simulink model "M10B39_es_V1"  (R2024b)
settings: Solver=ode23tb  StartTime=0.0  StopTime=20  FixedStep=0.001  RelTol=1e-3  EnableMultiTasking=on
InitFcn:
  | initAll;
values from neighbouring files (symbols this model uses):
  acom = 100    [initAll_V1.m]    (also in initAll_V2.m; initAll_V3.m; parameterinit.mat)
  AVm0 = [4.26082678503 4.656135219]    [parameterinit.mat]
  bcom = 50    [initAll_V1.m]    (also in initAll_V2.m; initAll_V3.m; parameterinit.mat)
  commun = 0*commun    [initAll_V1.m]    (also in initAll_V2.m; initAll_V3.m; parameterinit.mat = [0  0  0; 0  0  0; 0  0  0; 0  0  0])
  DataDelay = 0.0*DataDelay    [initAll_V1.m]    (also in initAll_V2.m; initAll_V3.m; parameterinit.mat = [0  0  0; 0  0  0; 0  0  0; 0  0  0])
  ESinit =     [parameterinit.mat]
  fB = 50    [initAll.m]    (also in initAll_V1.m; initAll_V2.m; initAll_V3.m; parameterinit.mat)
  Geninit = Generator_init(opdata,SynMach_in_gidx)    [initAll.m]    (also in initAll_V1.m; initAll_V2.m; initAll_V3.m = Generator_init(opdata_all,SynMach_in_gidx1); parameterinit.mat = )
  lam = 100    [initAll_V1.m]    (also in initAll_V2.m; initAll_V3.m; parameterinit.mat)
  SgridB = 100    [initAll.m]    (also in initAll_V1.m; initAll_V2.m; initAll_V3.m; parameterinit.mat)
  wB = 2*pi*fB    (= 314.159265359)    [initAll.m]    (also in initAll_V1.m; initAll_V2.m; initAll_V3.m; parameterinit.mat)
  Windinit =     [parameterinit.mat]
  YY_load = [3.65450097002 -2.05705688056 0 0 0 0 0 0 0 0 0 0 ... (1521 elements, 39x39)]    [parameterinit.mat]    (also in powerflowcaculate.m = full(YY))
undefined symbols (not defined in the file or in its folder): c1, c2, c3, c4, c5, c6, cp_nom, lambda_nom, P_wind_base, Pelec_base, Pnom
libraries: spsBistableLib x12, simulink_extras x4, slpidlib x1, simulink x1
(part 1 of 7)
settings Model: Creator=m  LastModifiedBy=86182
settings SolverCC: AlgebraicLoopSolver=TrustRegion
settings DataIOCC: SignalLoggingSaveFormat=ModelDataLogs  DSMLogging=off  ReturnWorkspaceOutputs=off  SignalLoggingName=logout
settings OptimizationCC: ExpressionDepthLimit=2147483647  LifeSpan=inf
settings DebuggingCC: SaveWithParameterizedLinksMsg=none  UnderspecifiedInitializationDetection=Classic  MergeDetectMultiDrivingBlocksExec=none  SignalResolutionControl=TryResolveAllWithWarning  MultiTaskDSMMsg=warning  MultiTaskCondExecSysMsg=none  FcnCallInpInsideContextMsg=warning  UnconnectedInputMsg=warning  UnconnectedOutputMsg=warning  UnconnectedLineMsg=warning  StateNameClashWarn=warning  SFUnexpectedBacktrackingDiag=warning  SFNoUnconditionalDefaultTransitionDiag=warning  SFExecutionAtInitializationDiag=none  ArithmeticOperatorsInVariantConditions=warning
settings HardwareCC: ProdBitPerPointer=32  ProdBitPerSizeT=32  ProdBitPerPtrDiffT=32  ProdLargestAtomicFloat=None  ProdIntDivRoundTo=Undefined  ProdEndianess=Unspecified  ProdWordSize=32  ProdHWDeviceType=32-bit Generic  TargetUnknown=on
settings ModelReferenceCC: EnableRefExpFcnMdlSchedulingChecks=on  PropagateSignalLabelsOutOfModel=off
settings SFSimCC: SimUseLocalCustomCode=off  CustomCodeUndefinedFunction=UseInterfaceOnly
settings RTWCC: RTWUseLocalCustomCode=off  GPUComputeCapability=3.5  DLArmComputeVersion=19.05
settings CodeAppCC: StateflowObjectComments=on
settings GRTTargetCC: TargetLangStandard=C89/C90 (ANSI)  CombineOutputUpdateFcns=off  GRTInterface=on
settings ConfigComp: CovMetricSettings=dw  CovSaveCumulativeToWorkspaceVar=on  CovSaveSingleToWorkspaceVar=on  CovExternalEMLEnable=off  CovSFcnEnable=off

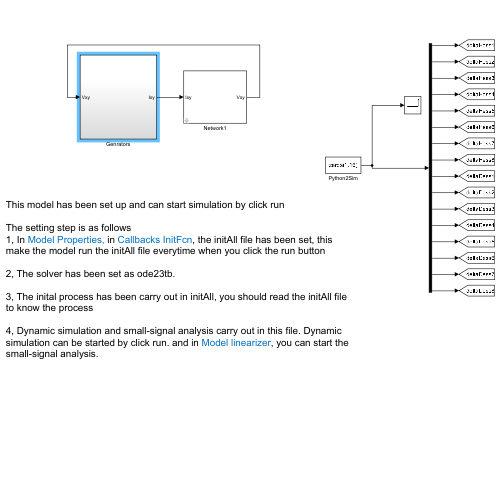
[thumbnail: Simulink's stored preview of the top-level diagram]
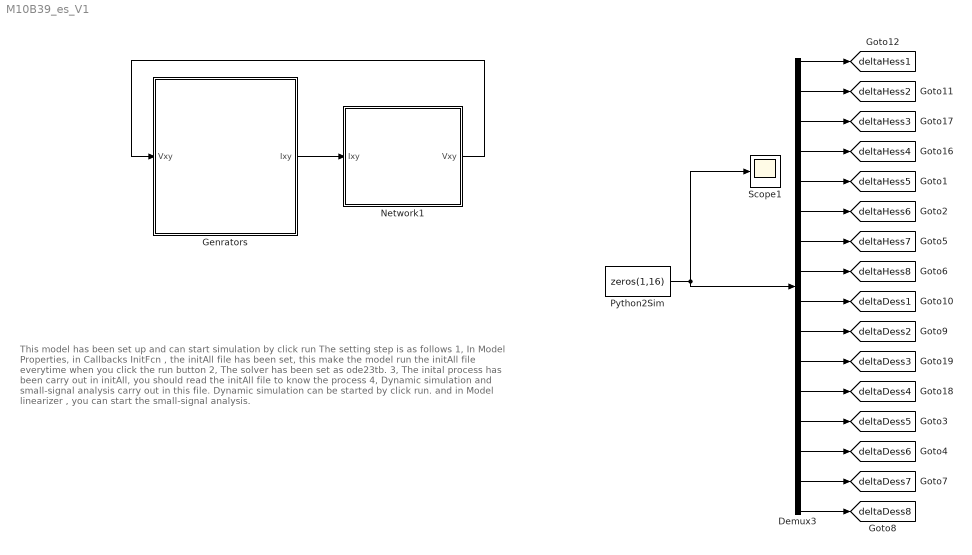
== system M10B39_es_V1 ==
  note: This model has been set up and can start simulation by click run
      |
      | The setting step is as follows
      | 1, In Model Properties, in Callbacks InitFcn , the initAll file has been set, this make the model run the initAll file everytime when you click the run button
      |
      | 2, The solver has been set as ode23tb.
      |
      | 3, The inital process has been carry out in initAll, you should read the initAll file to know the process
      |
      | 4, Dynamic simulation and small-signal analysis carry out in this file. Dynamic simulation can be started by click run. and in Model linearizer , you can start the small-signal analysis.
  Demux3 : Demux  Outputs=16
  Genrators : Subsystem
  Network1 : Subsystem  mask{YY_load=YY_load, ng=12, loadnode=31, loadsize=16}
  Python2Sim : Constant  Value=zeros(1,16)
  Scope1 : Scope
  tag scope: deltaDess1=global, deltaDess2=global, deltaDess3=global, deltaDess4=global, deltaDess5=global, deltaDess6=global, deltaDess7=global, deltaDess8=global, deltaHess1=global, deltaHess2=global, deltaHess3=global, deltaHess4=global, deltaHess5=global, deltaHess6=global, deltaHess7=global, deltaHess8=global
  wires:
  Genrators/1(Ixy) -> Network1/1(Ixy)
  Network1/1(Vxy) -> Genrators/1(Vxy)
  Demux3/3 -> [deltaHess3]
  Demux3/1 -> [deltaHess1]
  Demux3/2 -> [deltaHess2]
  Demux3/4 -> [deltaHess4]
  Demux3/9 -> [deltaDess1]
  Demux3/10 -> [deltaDess2]
  Demux3/11 -> [deltaDess3]
  Demux3/12 -> [deltaDess4]
  Demux3/5 -> [deltaHess5]
  Demux3/6 -> [deltaHess6]
  Demux3/13 -> [deltaDess5]
  Demux3/14 -> [deltaDess6]
  Demux3/7 -> [deltaHess7]
  Demux3/8 -> [deltaHess8]
  Demux3/15 -> [deltaDess7]
  Demux3/16 -> [deltaDess8]
  Python2Sim/1 -> Demux3/1, Scope1/1

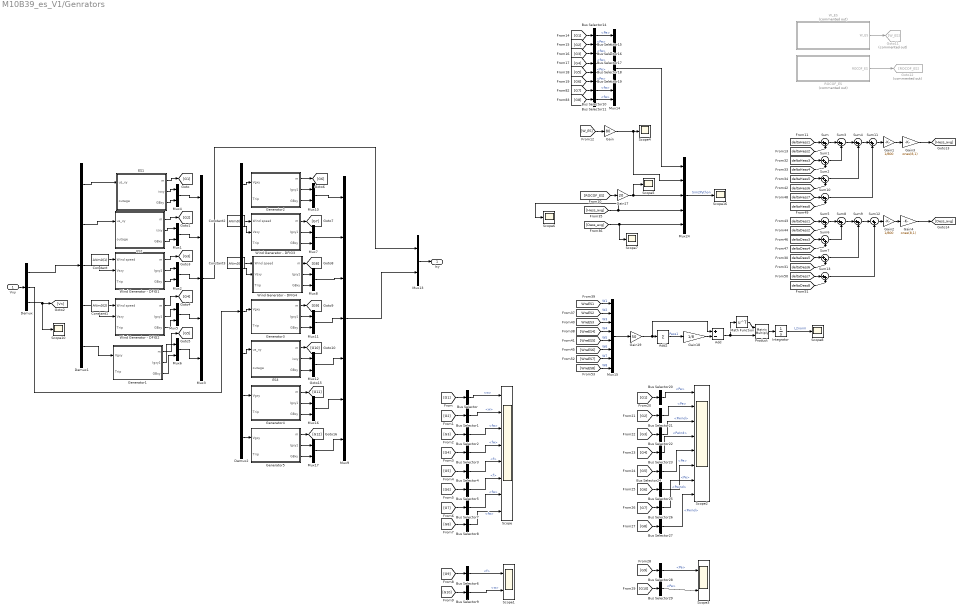
== system M10B39_es_V1/Genrators ==
  Vxy : Inport
  Add : Sum  Inputs=+-
  Add2 : Sum  Inputs=+
  Bus Selector : BusSelector  OutputSignals=w
  Bus Selector1 : BusSelector  OutputSignals=w
  Bus Selector{2..3,7..8,10..11,16..17} (8 alike) : BusSelector  OutputSignals=fw
  Bus Selector{14..15,18..21,24..25,28..29} (10 alike) : BusSelector  OutputSignals=Pe
  Bus Selector{22..23,26..27} (4 alike) : BusSelector  OutputSignals=Pwind
  Bus Selector4 : BusSelector  OutputSignals=f
  Bus Selector5 : BusSelector  OutputSignals=f
  Bus Selector6 : BusSelector  OutputSignals=f
  Bus Selector9 : BusSelector  OutputSignals=w
  Constant : Constant  Value=AVm0(1)
  Constant1 : Constant  Value=AVm0(2)
  Constant2 : Constant  Value=AVm0(3)
  Constant3 : Constant  Value=AVm0(4)
  Demux : Demux  Outputs=[10 14 27]
      settings: DisplayOption=none
  Demux1 : Demux  Outputs=5
      settings: DisplayOption=none
  Demux2 : Demux  Outputs=7
      settings: DisplayOption=none
  ES1 : Subsystem  mask{SvscB=ESinit.SvscBi(1), SgridB=SgridB, Kppll_VSC=ESinit.Kppll(1), Kipll_VSC=ESinit.Kipll(1), Dels_hvdc=ESinit.Dels_hvdc(1), Lpr=ESinit.Lpr(1), Rpr=ESinit.Rpr(1), wB=wB, Is_xA_0=ESinit.Isx0(1), Is_yA_0=ESinit.Isy0(1), KpP_VSC_A=ESinit.KpP(1), KiP_VSC_A=ESinit.KiP(1), KpId_VSC_A=ESinit.KpId(1), KiId_VSC_A=ESinit.KiId(1), KpQ_VSC_A=ESinit.KpQ(1), KiQ_VSC_A=ESinit.KiQ(1), KpIq_VSC_A=ESinit.KpIq(1), KiIq_VSC_A=ESinit.KiIq(1), Md_A_0=ESinit.Md0(1), Mq_A_0=ESinit.Mq0(1), Nd_A_0=ESinit.Nd0(1), Nq_A_0=ESinit.Nq0(1), KIR=ESinit.Kir(1), Kdroop=ESinit.Kdroop(1), Kdistributed=ESinit.Kdistributed(1), Kdistributed_d=ESinit.Kdistributed_d(1), Kpac_VSC_A=ESinit.Kpac(1), Kiac_VSC_A=ESinit.Kiac(1), P0=ESinit.P0(1), Q0=ESinit.Q0(1), usd0=ESinit.Usd0(1)}
      mask prompts: Kppll_VSC "Kppll"; Kipll_VSC "Kipll"; KpP_VSC_A "KpP"; KiP_VSC_A "KiP"; KpId_VSC_A "KpId"; KiId_VSC_A "KiId"; KpQ_VSC_A "KpQ"; KiQ_VSC_A "KiQ"; KpIq_VSC_A "KpIq"; KiIq_VSC_A "KiIq"; Kpac_VSC_A "Kpac"; Kiac_VSC_A "Kiac"
      mask DialogControl Container48 Prompt: Base value
      mask DialogControl Container7 Prompt: PLL
      mask DialogControl Container5 Prompt: Control parameter
      mask DialogControl Container8 Prompt: inital value
      mask DialogControl Container9 Prompt: AC side
      mask DialogControl Container10 Prompt: Parameter
      mask DialogControl Container11 Prompt: Initial value
      mask DialogControl Container18 Prompt: Control parameter
      mask DialogControl Container19 Prompt: d_axis_control parameter
      mask DialogControl Container23 Prompt: d_axis_control=1
      mask DialogControl Container26 Prompt: inner current control
      mask DialogControl Container21 Prompt: q_axis_control parameter
      mask DialogControl Container29 Prompt: q_axis_control=1
      mask DialogControl Container31 Prompt: inner current control
      mask DialogControl Container22 Prompt: inital value
      mask DialogControl Container35 Prompt: outer controller
      mask DialogControl Container36 Prompt: inner control
      mask DialogControl Container27 Prompt: Inertia control
      mask DialogControl Container28 Prompt: droop control
      mask DialogControl Container300 Prompt: distributed control
      mask DialogControl Container301 Prompt: Droop distributed control
      mask DialogControl Container40 Prompt: usdq_control
      mask DialogControl Container41 Prompt: PQinitial
      mask DialogControl Container42 Prompt: usd0initial
  ES2 : Subsystem  mask{SvscB=ESinit.SvscBi(2), SgridB=SgridB, Kppll_VSC=ESinit.Kppll(2), Kipll_VSC=ESinit.Kipll(2), Dels_hvdc=ESinit.Dels_hvdc(2), Lpr=ESinit.Lpr(2), Rpr=ESinit.Rpr(2), wB=wB, Is_xA_0=ESinit.Isx0(2), Is_yA_0=ESinit.Isy0(2), KpP_VSC_A=ESinit.KpP(2), KiP_VSC_A=ESinit.KiP(2), KpId_VSC_A=ESinit.KpId(2), KiId_VSC_A=ESinit.KiId(2), KpQ_VSC_A=ESinit.KpQ(2), KiQ_VSC_A=ESinit.KiQ(2), KpIq_VSC_A=ESinit.KpIq(2), KiIq_VSC_A=ESinit.KiIq(2), Md_A_0=ESinit.Md0(2), Mq_A_0=ESinit.Mq0(2), Nd_A_0=ESinit.Nd0(2), Nq_A_0=ESinit.Nq0(2), KIR=ESinit.Kir(2), Kdroop=ESinit.Kdroop(2), Kdistributed=ESinit.Kdistributed(2), Kdistributed_d=ESinit.Kdistributed_d(2), Kpac_VSC_A=ESinit.Kpac(2), Kiac_VSC_A=ESinit.Kiac(2), P0=ESinit.P0(2), Q0=ESinit.Q0(2), usd0=ESinit.Usd0(2)}
      mask prompts: Kppll_VSC "Kppll"; Kipll_VSC "Kipll"; KpP_VSC_A "KpP"; KiP_VSC_A "KiP"; KpId_VSC_A "KpId"; KiId_VSC_A "KiId"; KpQ_VSC_A "KpQ"; KiQ_VSC_A "KiQ"; KpIq_VSC_A "KpIq"; KiIq_VSC_A "KiIq"; Kpac_VSC_A "Kpac"; Kiac_VSC_A "Kiac"
      mask DialogControl Container48 Prompt: Base value
      mask DialogControl Container7 Prompt: PLL
      mask DialogControl Container5 Prompt: Control parameter
      mask DialogControl Container8 Prompt: inital value
      mask DialogControl Container9 Prompt: AC side
      mask DialogControl Container10 Prompt: Parameter
      mask DialogControl Container11 Prompt: Initial value
      mask DialogControl Container18 Prompt: Control parameter
      mask DialogControl Container19 Prompt: d_axis_control parameter
      mask DialogControl Container23 Prompt: d_axis_control=1
      mask DialogControl Container26 Prompt: inner current control
      mask DialogControl Container21 Prompt: q_axis_control parameter
      mask DialogControl Container29 Prompt: q_axis_control=1
      mask DialogControl Container31 Prompt: inner current control
      mask DialogControl Container22 Prompt: inital value
      mask DialogControl Container35 Prompt: outer controller
      mask DialogControl Container36 Prompt: inner control
      mask DialogControl Container27 Prompt: Inertia control
      mask DialogControl Container28 Prompt: droop control
      mask DialogControl Container300 Prompt: distributed control
      mask DialogControl Container301 Prompt: Droop distributed control
      mask DialogControl Container40 Prompt: usdq_control
      mask DialogControl Container41 Prompt: PQinitial
      mask DialogControl Container42 Prompt: usd0initial
  ES3 : Subsystem  mask{SvscB=ESinit.SvscBi(3), SgridB=SgridB, Kppll_VSC=ESinit.Kppll(3), Kipll_VSC=ESinit.Kipll(3), Dels_hvdc=ESinit.Dels_hvdc(3), Lpr=ESinit.Lpr(3), Rpr=ESinit.Rpr(3), wB=wB, Is_xA_0=ESinit.Isx0(3), Is_yA_0=ESinit.Isy0(3), KpP_VSC_A=ESinit.KpP(3), KiP_VSC_A=ESinit.KiP(3), KpId_VSC_A=ESinit.KpId(3), KiId_VSC_A=ESinit.KiId(3), KpQ_VSC_A=ESinit.KpQ(3), KiQ_VSC_A=ESinit.KiQ(3), KpIq_VSC_A=ESinit.KpIq(3), KiIq_VSC_A=ESinit.KiIq(3), Md_A_0=ESinit.Md0(3), Mq_A_0=ESinit.Mq0(3), Nd_A_0=ESinit.Nd0(3), Nq_A_0=ESinit.Nq0(3), KIR=ESinit.Kir(3), Kdroop=ESinit.Kdroop(3), Kdistributed=ESinit.Kdistributed(3), Kdistributed_d=ESinit.Kdistributed_d(3), Kpac_VSC_A=ESinit.Kpac(3), Kiac_VSC_A=ESinit.Kiac(3), P0=ESinit.P0(3), Q0=ESinit.Q0(3), usd0=ESinit.Usd0(3)}
      mask prompts: Kppll_VSC "Kppll"; Kipll_VSC "Kipll"; KpP_VSC_A "KpP"; KiP_VSC_A "KiP"; KpId_VSC_A "KpId"; KiId_VSC_A "KiId"; KpQ_VSC_A "KpQ"; KiQ_VSC_A "KiQ"; KpIq_VSC_A "KpIq"; KiIq_VSC_A "KiIq"; Kpac_VSC_A "Kpac"; Kiac_VSC_A "Kiac"
      mask DialogControl Container48 Prompt: Base value
      mask DialogControl Container7 Prompt: PLL
      mask DialogControl Container5 Prompt: Control parameter
      mask DialogControl Container8 Prompt: inital value
      mask DialogControl Container9 Prompt: AC side
      mask DialogControl Container10 Prompt: Parameter
      mask DialogControl Container11 Prompt: Initial value
      mask DialogControl Container18 Prompt: Control parameter
      mask DialogControl Container19 Prompt: d_axis_control parameter
      mask DialogControl Container23 Prompt: d_axis_control=1
      mask DialogControl Container26 Prompt: inner current control
      mask DialogControl Container21 Prompt: q_axis_control parameter
      mask DialogControl Container29 Prompt: q_axis_control=1
      mask DialogControl Container31 Prompt: inner current control
      mask DialogControl Container22 Prompt: inital value
      mask DialogControl Container35 Prompt: outer controller
      mask DialogControl Container36 Prompt: inner control
      mask DialogControl Container27 Prompt: Inertia control
      mask DialogControl Container28 Prompt: droop control
      mask DialogControl Container300 Prompt: distributed control
      mask DialogControl Container301 Prompt: Droop distributed control
      mask DialogControl Container40 Prompt: usdq_control
      mask DialogControl Container41 Prompt: PQinitial
      mask DialogControl Container42 Prompt: usd0initial
  Gain : Gain  Gain=80
  Gain1 : Gain  Gain=1/800
  Gain17 : Gain  Gain=20
  Gain18 : Gain  Gain=1/8
  Gain19 : Gain  Gain=50
  Gain2 : Gain  Gain=1/800
  Gain3 : Gain  Gain=ones(8,1)
  Gain4 : Gain  Gain=ones(8,1)
  Generator1 : Subsystem  mask{wB=wB, SgenB=Geninit.SgenB(1), SgridB=SgridB, Xq=Geninit.Xq(1), Xq1=Geninit.Xq1(1), Xq11=Geninit.Xq11(1), Tq0=Geninit.Tq0(1), Tq10=Geninit.Tq10(1), Eq10=Geninit.Eq1(1), Eq110=Geninit.Eq11(1), Xd=Geninit.Xd(1), Xd1=Geninit.Xd1(1), Xd11=Geninit.Xd11(1), Td0=Geninit.Td0(1), Td10=Geninit.Td10(1), Ed10=Geninit.Ed1(1), Ed110=Geninit.Ed11(1), H=Geninit.Tj(1), D=Geninit.D(1), delta0=Geninit.Delta(1), w0=1, Pm0=Geninit.Pm0(1), Ka=Geninit.Ka(1), Tb=Geninit.Tb(1), Tc=Geninit.Tc(1), Efmax=Geninit.Efmax(1), Efmin=Geninit.Efmin(1), Vref=Geninit.Vref(1), Ef10=Geninit.Vf1(1), S_PSS=Geninit.EnablePSS(1), Kpss=Geninit.kpss(1), Tw_P=Geninit.Tw_P(1), T1_P=Geninit.T1_P(1), T2_P=Geninit.T2_P(1), T3_P=Geninit.T3_P(1), T4_P=Geninit.T4_P(1), Upmax=Geninit.Upmax(1), Upmin=Geninit.Upmin(1), S_Gov=Geninit.Enablegov(1), a_G=Geninit.a_G(1), b_G=Geninit.b_G(1), Tg_G=Geninit.Tg_G(1), dPmax=Geninit.dPmax(1), dPmin=Geninit.dPmin(1)}
      mask prompts: S_PSS "Enable PSS"; Tw_P "Tw"; T1_P "T1"; T2_P "T2"; T3_P "T3"; T4_P "T4"; S_Gov "Enable Governor"; a_G "a"; b_G "b"; Tg_G "Tg"
      mask help: This is a six-order synchronous generator with exciter system, governor and PSS.
      mask DialogControl Container6 Prompt: Machine parameter
      mask DialogControl Container3 Prompt: q axis parameter
      mask DialogControl ParameterGroupVar Prompt: d axis parameter
      mask DialogControl Container4 Prompt: machine parameter
      mask DialogControl Container12 Prompt: Excitation System parameter
      mask DialogControl Container20 Prompt: parameter
      mask DialogControl Container21 Prompt: inital value
      mask DialogControl Container10 Prompt: PSS parameter
      mask DialogControl Container13 Prompt: Governor parameter
  Generator2 : Subsystem  mask{wB=wB, SgenB=Geninit.SgenB(2), SgridB=SgridB, Xq=Geninit.Xq(2), Xq1=Geninit.Xq1(2), Xq11=Geninit.Xq11(2), Tq0=Geninit.Tq0(2), Tq10=Geninit.Tq10(2), Eq10=Geninit.Eq1(2), Eq110=Geninit.Eq11(2), Xd=Geninit.Xd(2), Xd1=Geninit.Xd1(2), Xd11=Geninit.Xd11(2), Td0=Geninit.Td0(2), Td10=Geninit.Td10(2), Ed10=Geninit.Ed1(2), Ed110=Geninit.Ed11(2), H=Geninit.Tj(2), D=Geninit.D(2), delta0=Geninit.Delta(2), w0=1, Pm0=Geninit.Pm0(2), Ka=Geninit.Ka(2), Tb=Geninit.Tb(2), Tc=Geninit.Tc(2), Efmax=Geninit.Efmax(2), Efmin=Geninit.Efmin(2), Vref=Geninit.Vref(2), Ef10=Geninit.Vf1(2), S_PSS=Geninit.EnablePSS(2), Kpss=Geninit.kpss(2), Tw_P=Geninit.Tw_P(2), T1_P=Geninit.T1_P(2), T2_P=Geninit.T2_P(2), T3_P=Geninit.T3_P(2), T4_P=Geninit.T4_P(2), Upmax=Geninit.Upmax(2), Upmin=Geninit.Upmin(2), S_Gov=Geninit.Enablegov(2), a_G=Geninit.a_G(2), b_G=Geninit.b_G(2), Tg_G=Geninit.Tg_G(2), dPmax=Geninit.dPmax(2), dPmin=Geninit.dPmin(2)}
      mask prompts: S_PSS "Enable PSS"; Tw_P "Tw"; T1_P "T1"; T2_P "T2"; T3_P "T3"; T4_P "T4"; S_Gov "Enable Governor"; a_G "a"; b_G "b"; Tg_G "Tg"
      mask help: This is a six-order synchronous generator with exciter system, governor and PSS.
      mask DialogControl Container6 Prompt: Machine parameter
      mask DialogControl Container3 Prompt: q axis parameter
      mask DialogControl ParameterGroupVar Prompt: d axis parameter
      mask DialogControl Container4 Prompt: machine parameter
      mask DialogControl Container12 Prompt: Excitation System parameter
      mask DialogControl Container20 Prompt: parameter
      mask DialogControl Container21 Prompt: inital value
      mask DialogControl Container10 Prompt: PSS parameter
      mask DialogControl Container13 Prompt: Governor parameter
  Generator3 : Subsystem  mask{wB=wB, SgenB=Geninit.SgenB(3), SgridB=SgridB, Xq=Geninit.Xq(3), Xq1=Geninit.Xq1(3), Xq11=Geninit.Xq11(3), Tq0=Geninit.Tq0(3), Tq10=Geninit.Tq10(3), Eq10=Geninit.Eq1(3), Eq110=Geninit.Eq11(3), Xd=Geninit.Xd(3), Xd1=Geninit.Xd1(3), Xd11=Geninit.Xd11(3), Td0=Geninit.Td0(3), Td10=Geninit.Td10(3), Ed10=Geninit.Ed1(3), Ed110=Geninit.Ed11(3), H=Geninit.Tj(3), D=Geninit.D(3), delta0=Geninit.Delta(3), w0=1, Pm0=Geninit.Pm0(3), Ka=Geninit.Ka(3), Tb=Geninit.Tb(3), Tc=Geninit.Tc(3), Efmax=Geninit.Efmax(3), Efmin=Geninit.Efmin(3), Vref=Geninit.Vref(3), Ef10=Geninit.Vf1(3), S_PSS=Geninit.EnablePSS(3), Kpss=Geninit.kpss(3), Tw_P=Geninit.Tw_P(3), T1_P=Geninit.T1_P(3), T2_P=Geninit.T2_P(3), T3_P=Geninit.T3_P(3), T4_P=Geninit.T4_P(3), Upmax=Geninit.Upmax(3), Upmin=Geninit.Upmin(3), S_Gov=Geninit.Enablegov(3), a_G=Geninit.a_G(3), b_G=Geninit.b_G(3), Tg_G=Geninit.Tg_G(3), dPmax=Geninit.dPmax(3), dPmin=Geninit.dPmin(3)}
      mask prompts: S_PSS "Enable PSS"; Tw_P "Tw"; T1_P "T1"; T2_P "T2"; T3_P "T3"; T4_P "T4"; S_Gov "Enable Governor"; a_G "a"; b_G "b"; Tg_G "Tg"
      mask help: This is a six-order synchronous generator with exciter system, governor and PSS.
      mask DialogControl Container6 Prompt: Machine parameter
      mask DialogControl Container3 Prompt: q axis parameter
      mask DialogControl ParameterGroupVar Prompt: d axis parameter
      mask DialogControl Container4 Prompt: machine parameter
      mask DialogControl Container12 Prompt: Excitation System parameter
      mask DialogControl Container20 Prompt: parameter
      mask DialogControl Container21 Prompt: inital value
      mask DialogControl Container10 Prompt: PSS parameter
      mask DialogControl Container13 Prompt: Governor parameter
  Generator4 : Subsystem  mask{wB=wB, SgenB=Geninit.SgenB(4), SgridB=SgridB, Xq=Geninit.Xq(4), Xq1=Geninit.Xq1(4), Xq11=Geninit.Xq11(4), Tq0=Geninit.Tq0(4), Tq10=Geninit.Tq10(4), Eq10=Geninit.Eq1(4), Eq110=Geninit.Eq11(4), Xd=Geninit.Xd(4), Xd1=Geninit.Xd1(4), Xd11=Geninit.Xd11(4), Td0=Geninit.Td0(4), Td10=Geninit.Td10(4), Ed10=Geninit.Ed1(4), Ed110=Geninit.Ed11(4), H=Geninit.Tj(4), D=Geninit.D(4), delta0=Geninit.Delta(4), w0=1, Pm0=Geninit.Pm0(4), Ka=Geninit.Ka(4), Tb=Geninit.Tb(4), Tc=Geninit.Tc(4), Efmax=Geninit.Efmax(4), Efmin=Geninit.Efmin(4), Vref=Geninit.Vref(4), Ef10=Geninit.Vf1(4), S_PSS=Geninit.EnablePSS(4), Kpss=Geninit.kpss(4), Tw_P=Geninit.Tw_P(4), T1_P=Geninit.T1_P(4), T2_P=Geninit.T2_P(4), T3_P=Geninit.T3_P(4), T4_P=Geninit.T4_P(4), Upmax=Geninit.Upmax(4), Upmin=Geninit.Upmin(4), S_Gov=Geninit.Enablegov(4), a_G=Geninit.a_G(4), b_G=Geninit.b_G(4), Tg_G=Geninit.Tg_G(4), dPmax=Geninit.dPmax(4), dPmin=Geninit.dPmin(4)}
      mask prompts: S_PSS "Enable PSS"; Tw_P "Tw"; T1_P "T1"; T2_P "T2"; T3_P "T3"; T4_P "T4"; S_Gov "Enable Governor"; a_G "a"; b_G "b"; Tg_G "Tg"
      mask help: This is a six-order synchronous generator with exciter system, governor and PSS.
      mask DialogControl Container6 Prompt: Machine parameter
      mask DialogControl Container3 Prompt: q axis parameter
      mask DialogControl ParameterGroupVar Prompt: d axis parameter
      mask DialogControl Container4 Prompt: machine parameter
      mask DialogControl Container12 Prompt: Excitation System parameter
      mask DialogControl Container20 Prompt: parameter
      mask DialogControl Container21 Prompt: inital value
      mask DialogControl Container10 Prompt: PSS parameter
      mask DialogControl Container13 Prompt: Governor parameter
  Generator5 : Subsystem  mask{wB=wB, SgenB=Geninit.SgenB(5), SgridB=SgridB, Xq=Geninit.Xq(5), Xq1=Geninit.Xq1(5), Xq11=Geninit.Xq11(5), Tq0=Geninit.Tq0(5), Tq10=Geninit.Tq10(5), Eq10=Geninit.Eq1(5), Eq110=Geninit.Eq11(5), Xd=Geninit.Xd(5), Xd1=Geninit.Xd1(5), Xd11=Geninit.Xd11(5), Td0=Geninit.Td0(5), Td10=Geninit.Td10(5), Ed10=Geninit.Ed1(5), Ed110=Geninit.Ed11(5), H=Geninit.Tj(5), D=Geninit.D(5), delta0=Geninit.Delta(5), w0=1, Pm0=Geninit.Pm0(5), Ka=Geninit.Ka(5), Tb=Geninit.Tb(5), Tc=Geninit.Tc(5), Efmax=Geninit.Efmax(5), Efmin=Geninit.Efmin(5), Vref=Geninit.Vref(5), Ef10=Geninit.Vf1(5), S_PSS=Geninit.EnablePSS(5), Kpss=Geninit.kpss(5), Tw_P=Geninit.Tw_P(5), T1_P=Geninit.T1_P(5), T2_P=Geninit.T2_P(5), T3_P=Geninit.T3_P(5), T4_P=Geninit.T4_P(5), Upmax=Geninit.Upmax(5), Upmin=Geninit.Upmin(5), S_Gov=Geninit.Enablegov(5), a_G=Geninit.a_G(5), b_G=Geninit.b_G(5), Tg_G=Geninit.Tg_G(5), dPmax=Geninit.dPmax(5), dPmin=Geninit.dPmin(5)}
      mask prompts: S_PSS "Enable PSS"; Tw_P "Tw"; T1_P "T1"; T2_P "T2"; T3_P "T3"; T4_P "T4"; S_Gov "Enable Governor"; a_G "a"; b_G "b"; Tg_G "Tg"
      mask help: This is a six-order synchronous generator with exciter system, governor and PSS.
      mask DialogControl Container6 Prompt: Machine parameter
      mask DialogControl Container3 Prompt: q axis parameter
      mask DialogControl ParameterGroupVar Prompt: d axis parameter
      mask DialogControl Container4 Prompt: machine parameter
      mask DialogControl Container12 Prompt: Excitation System parameter
      mask DialogControl Container20 Prompt: parameter
      mask DialogControl Container21 Prompt: inital value
      mask DialogControl Container10 Prompt: PSS parameter
      mask DialogControl Container13 Prompt: Governor parameter
  Goto11 : Goto  Commented=on  GotoTag=W_ES
  Goto12 : Goto  Commented=on  GotoTag=ROCOF_ES
  Integrator : Integrator
  Math Function : Math  Operator=transpose
  Mux{1..2,4..8,10..13,16..17} (13 alike) : Mux  Inputs=2
  Mux14 : Mux  Inputs=8
  Mux15 : Mux  Inputs=8
  Mux24 : Mux  Inputs=5
  Mux3 : Mux  Inputs=5
  Mux9 : Mux  Inputs=7
  Product : Product  Multiplication=Matrix(*)
  ROCOF_ES : Subsystem  Commented=on
  Scope : Scope  NumInputPorts=8
  Scope1 : Scope  NumInputPorts=2
  Scope{4..8,10,16} (7 alike) : Scope
  Scope2 : Scope  NumInputPorts=8
  Scope3 : Scope  NumInputPorts=2
  Sum{,1..13} (14 alike) : Sum  Inputs=|++
  W_ES : Subsystem  Commented=on
  Wind Generator - DFIG1 : Subsystem  mask{NN=Windinit.NN(1), SwgBi=Windinit.SwgBi(1), SmecBi=100, SgridB=SgridB, Atheta=Windinit.Atheta(1), Kppll=Windinit.Kppll_wind(1), Kipll=Windinit.Kipll_wind(1), pitch=[500 45 2], Srotors=1.3, H=Windinit.H(1), Wr0=Windinit.Wr0(1), Xa=Windinit.Xa(1), Xa1=Windinit.Xa1(1), Lm=Windinit.Lm(1), Lr=Windinit.Lr(1), Rs=Windinit.Rs(1), Ls=Windinit.Ls(1), Ta0=Windinit.Ta0(1), NPf=Windinit.NPf(1), Za=Windinit.Za{1}, Ex0=Windinit.Ex_ref(1), Ey0=Windinit.Ey_ref(1), wB=wB, KpP_rw=Windinit.KpP_rw(1), KiP_rw=Windinit.KiP_rw(1), KpId_rw=Windinit.KpId_rw(1), KiId_rw=Windinit.KiId_rw(1), KpQ_rw=Windinit.KpQ_rw(1), KiQ_rw=Windinit.KiQ_rw(1), KpIq_rw=Windinit.KpIq_rw(1), KiIq_rw=Windinit.KiIq_rw(1), Ird_ref=Windinit.Ird_ref(1), Irq_ref=Windinit.Irq_ref(1), Qs0=Windinit.Qs0(1), KpDC_gw=Windinit.KpDC_gw(1), KiDC_gw=Windinit.KiDC_gw(1), KpId_gw=Windinit.KpId_gw(1), KiId_gw=Windinit.KiId_gw(1), KpIq_gw=Windinit.KpIq_gw(1), KiIq_gw=Windinit.KiIq_gw(1), Vdc_w=Windinit.Vdc_w(1), Icd_ref=Windinit.Icd_ref(1), Icq_ref=Windinit.Icq_ref(1), Vcd_ref=Windinit.Vcd_ref(1), Vcq_ref=Windinit.Vcq_ref(1), Lg=Windinit.Lg(1), Rg=Windinit.Rg(1), Icx0=Windinit.Icx0(1), Icy0=Windinit.Icy0(1), C_w=Windinit.C_w(1), Vdc0=Windinit.Vdc0(1)}
      mask prompts: pitch "pitch_gain，pitch_max，pitch_rate"; Srotors "Start Rotor Speed"; Ex0 "Ex"; Ey0 "Ey"
      mask init:
      | pitch_gain=pitch(1);
      | pitch_max=pitch(2);
      | pitch_rate=pitch(3);
      | 
      | %该风机模型的基准容量
      | 
      | SwgeqB=SwgBi.*NN;
      mask DialogControl Container4 Prompt: PLL/Wind turbine
      mask DialogControl Container31 Prompt: Base value
      mask DialogControl Container23 Prompt: PLL
      mask DialogControl Container6 Prompt: inital value
      mask DialogControl Container5 Prompt: PI parameter
      mask DialogControl Container24 Prompt: Wind turbine
      mask DialogControl Container25 Prompt: pitch control
      mask DialogControl Container7 Prompt: Machine parameter
      mask DialogControl Container8 Prompt: Rotor
      mask DialogControl Container9 Prompt: Machine
      mask DialogControl Container10 Prompt: parameter
      mask DialogControl Container11 Prompt: inital value
      mask DialogControl Container12 Prompt: Rotor side control
      mask DialogControl Container13 Prompt: Control parameter
      mask DialogControl Container14 Prompt: Initial value
      mask DialogControl Container15 Prompt: reactive power
      mask DialogControl Container16 Prompt: Grid side control
      mask DialogControl Container17 Prompt: parameter
      mask DialogControl Container18 Prompt: reference
      mask DialogControl Container19 Prompt: inital value
      mask DialogControl Container20 Prompt: converter function
      mask DialogControl Container21 Prompt: inital value
      mask DialogControl Container22 Prompt: DC function
  Wind Generator - DFIG2 : Subsystem  mask{NN=Windinit.NN(2), SwgBi=Windinit.SwgBi(2), SmecBi=100, SgridB=SgridB, Atheta=Windinit.Atheta(2), Kppll=Windinit.Kppll_wind(2), Kipll=Windinit.Kipll_wind(2), pitch=[500 45 2], Srotors=1.3, H=Windinit.H(2), Wr0=Windinit.Wr0(2), Xa=Windinit.Xa(2), Xa1=Windinit.Xa1(2), Lm=Windinit.Lm(2), Lr=Windinit.Lr(2), Rs=Windinit.Rs(2), Ls=Windinit.Ls(2), Ta0=Windinit.Ta0(2), NPf=Windinit.NPf(2), Za=Windinit.Za{2}, Ex0=Windinit.Ex_ref(2), Ey0=Windinit.Ey_ref(2), wB=wB, KpP_rw=Windinit.KpP_rw(2), KiP_rw=Windinit.KiP_rw(2), KpId_rw=Windinit.KpId_rw(2), KiId_rw=Windinit.KiId_rw(2), KpQ_rw=Windinit.KpQ_rw(2), KiQ_rw=Windinit.KiQ_rw(2), KpIq_rw=Windinit.KpIq_rw(2), KiIq_rw=Windinit.KiIq_rw(2), Ird_ref=Windinit.Ird_ref(2), Irq_ref=Windinit.Irq_ref(2), Qs0=Windinit.Qs0(2), KpDC_gw=Windinit.KpDC_gw(2), KiDC_gw=Windinit.KiDC_gw(2), KpId_gw=Windinit.KpId_gw(2), KiId_gw=Windinit.KiId_gw(2), KpIq_gw=Windinit.KpIq_gw(2), KiIq_gw=Windinit.KiIq_gw(2), Vdc_w=Windinit.Vdc_w(2), Icd_ref=Windinit.Icd_ref(2), Icq_ref=Windinit.Icq_ref(2), Vcd_ref=Windinit.Vcd_ref(2), Vcq_ref=Windinit.Vcq_ref(2), Lg=Windinit.Lg(2), Rg=Windinit.Rg(2), Icx0=Windinit.Icx0(2), Icy0=Windinit.Icy0(2), C_w=Windinit.C_w(2), Vdc0=Windinit.Vdc0(2)}
      mask prompts: pitch "pitch_gain，pitch_max，pitch_rate"; Srotors "Start Rotor Speed"; Ex0 "Ex"; Ey0 "Ey"
      mask init:
      | pitch_gain=pitch(1);
      | pitch_max=pitch(2);
      | pitch_rate=pitch(3);
      | 
      | %该风机模型的基准容量
      | 
      | SwgeqB=SwgBi.*NN;
      mask DialogControl Container4 Prompt: PLL/Wind turbine
      mask DialogControl Container31 Prompt: Base value
      mask DialogControl Container23 Prompt: PLL
      mask DialogControl Container6 Prompt: inital value
      mask DialogControl Container5 Prompt: PI parameter
      mask DialogControl Container24 Prompt: Wind turbine
      mask DialogControl Container25 Prompt: pitch control
      mask DialogControl Container7 Prompt: Machine parameter
      mask DialogControl Container8 Prompt: Rotor
      mask DialogControl Container9 Prompt: Machine
      mask DialogControl Container10 Prompt: parameter
      mask DialogControl Container11 Prompt: inital value
      mask DialogControl Container12 Prompt: Rotor side control
      mask DialogControl Container13 Prompt: Control parameter
      mask DialogControl Container14 Prompt: Initial value
      mask DialogControl Container15 Prompt: reactive power
      mask DialogControl Container16 Prompt: Grid side control
      mask DialogControl Container17 Prompt: parameter
      mask DialogControl Container18 Prompt: reference
      mask DialogControl Container19 Prompt: inital value
      mask DialogControl Container20 Prompt: converter function
      mask DialogControl Container21 Prompt: inital value
      mask DialogControl Container22 Prompt: DC function
  Wind Generator - DFIG3 : Subsystem  mask{NN=Windinit.NN(3), SwgBi=Windinit.SwgBi(3), SmecBi=100, SgridB=SgridB, Atheta=Windinit.Atheta(3), Kppll=Windinit.Kppll_wind(3), Kipll=Windinit.Kipll_wind(3), pitch=[500 45 2], Srotors=1.3, H=Windinit.H(3), Wr0=Windinit.Wr0(3), Xa=Windinit.Xa(3), Xa1=Windinit.Xa1(3), Lm=Windinit.Lm(3), Lr=Windinit.Lr(3), Rs=Windinit.Rs(3), Ls=Windinit.Ls(3), Ta0=Windinit.Ta0(3), NPf=Windinit.NPf(3), Za=Windinit.Za{3}, Ex0=Windinit.Ex_ref(3), Ey0=Windinit.Ey_ref(3), wB=wB, KpP_rw=Windinit.KpP_rw(3), KiP_rw=Windinit.KiP_rw(3), KpId_rw=Windinit.KpId_rw(3), KiId_rw=Windinit.KiId_rw(3), KpQ_rw=Windinit.KpQ_rw(3), KiQ_rw=Windinit.KiQ_rw(3), KpIq_rw=Windinit.KpIq_rw(3), KiIq_rw=Windinit.KiIq_rw(3), Ird_ref=Windinit.Ird_ref(3), Irq_ref=Windinit.Irq_ref(3), Qs0=Windinit.Qs0(3), KpDC_gw=Windinit.KpDC_gw(3), KiDC_gw=Windinit.KiDC_gw(3), KpId_gw=Windinit.KpId_gw(3), KiId_gw=Windinit.KiId_gw(3), KpIq_gw=Windinit.KpIq_gw(3), KiIq_gw=Windinit.KiIq_gw(3), Vdc_w=Windinit.Vdc_w(3), Icd_ref=Windinit.Icd_ref(3), Icq_ref=Windinit.Icq_ref(3), Vcd_ref=Windinit.Vcd_ref(3), Vcq_ref=Windinit.Vcq_ref(3), Lg=Windinit.Lg(3), Rg=Windinit.Rg(3), Icx0=Windinit.Icx0(3), Icy0=Windinit.Icy0(3), C_w=Windinit.C_w(3), Vdc0=Windinit.Vdc0(3)}
      mask prompts: pitch "pitch_gain，pitch_max，pitch_rate"; Srotors "Start Rotor Speed"; Ex0 "Ex"; Ey0 "Ey"
      mask init:
      | pitch_gain=pitch(1);
      | pitch_max=pitch(2);
      | pitch_rate=pitch(3);
      | 
      | %该风机模型的基准容量
      | 
      | SwgeqB=SwgBi.*NN;
      mask DialogControl Container4 Prompt: PLL/Wind turbine
      mask DialogControl Container31 Prompt: Base value
      mask DialogControl Container23 Prompt: PLL
      mask DialogControl Container6 Prompt: inital value
      mask DialogControl Container5 Prompt: PI parameter
      mask DialogControl Container24 Prompt: Wind turbine
      mask DialogControl Container25 Prompt: pitch control
      mask DialogControl Container7 Prompt: Machine parameter
      mask DialogControl Container8 Prompt: Rotor
      mask DialogControl Container9 Prompt: Machine
      mask DialogControl Container10 Prompt: parameter
      mask DialogControl Container11 Prompt: inital value
      mask DialogControl Container12 Prompt: Rotor side control
      mask DialogControl Container13 Prompt: Control parameter
      mask DialogControl Container14 Prompt: Initial value
      mask DialogControl Container15 Prompt: reactive power
      mask DialogControl Container16 Prompt: Grid side control
      mask DialogControl Container17 Prompt: parameter
      mask DialogControl Container18 Prompt: reference
      mask DialogControl Container19 Prompt: inital value
      mask DialogControl Container20 Prompt: converter function
      mask DialogControl Container21 Prompt: inital value
      mask DialogControl Container22 Prompt: DC function
  Wind Generator - DFIG4 : Subsystem  mask{NN=Windinit.NN(4), SwgBi=Windinit.SwgBi(4), SmecBi=100, SgridB=SgridB, Atheta=Windinit.Atheta(4), Kppll=Windinit.Kppll_wind(4), Kipll=Windinit.Kipll_wind(4), pitch=[500 45 2], Srotors=1.3, H=Windinit.H(4), Wr0=Windinit.Wr0(4), Xa=Windinit.Xa(4), Xa1=Windinit.Xa1(4), Lm=Windinit.Lm(4), Lr=Windinit.Lr(4), Rs=Windinit.Rs(4), Ls=Windinit.Ls(4), Ta0=Windinit.Ta0(4), NPf=Windinit.NPf(4), Za=Windinit.Za{4}, Ex0=Windinit.Ex_ref(4), Ey0=Windinit.Ey_ref(4), wB=wB, KpP_rw=Windinit.KpP_rw(4), KiP_rw=Windinit.KiP_rw(4), KpId_rw=Windinit.KpId_rw(4), KiId_rw=Windinit.KiId_rw(4), KpQ_rw=Windinit.KpQ_rw(4), KiQ_rw=Windinit.KiQ_rw(4), KpIq_rw=Windinit.KpIq_rw(4), KiIq_rw=Windinit.KiIq_rw(4), Ird_ref=Windinit.Ird_ref(4), Irq_ref=Windinit.Irq_ref(4), Qs0=Windinit.Qs0(4), KpDC_gw=Windinit.KpDC_gw(4), KiDC_gw=Windinit.KiDC_gw(4), KpId_gw=Windinit.KpId_gw(4), KiId_gw=Windinit.KiId_gw(4), KpIq_gw=Windinit.KpIq_gw(4), KiIq_gw=Windinit.KiIq_gw(4), Vdc_w=Windinit.Vdc_w(4), Icd_ref=Windinit.Icd_ref(4), Icq_ref=Windinit.Icq_ref(4), Vcd_ref=Windinit.Vcd_ref(4), Vcq_ref=Windinit.Vcq_ref(4), Lg=Windinit.Lg(4), Rg=Windinit.Rg(4), Icx0=Windinit.Icx0(4), Icy0=Windinit.Icy0(4), C_w=Windinit.C_w(4), Vdc0=Windinit.Vdc0(4)}
      mask prompts: pitch "pitch_gain，pitch_max，pitch_rate"; Srotors "Start Rotor Speed"; Ex0 "Ex"; Ey0 "Ey"
      mask init:
      | pitch_gain=pitch(1);
      | pitch_max=pitch(2);
      | pitch_rate=pitch(3);
      | 
      | %该风机模型的基准容量
      | 
      | SwgeqB=SwgBi.*NN;
      mask DialogControl Container4 Prompt: PLL/Wind turbine
      mask DialogControl Container31 Prompt: Base value
      mask DialogControl Container23 Prompt: PLL
      mask DialogControl Container6 Prompt: inital value
      mask DialogControl Container5 Prompt: PI parameter
      mask DialogControl Container24 Prompt: Wind turbine
      mask DialogControl Container25 Prompt: pitch control
      mask DialogControl Container7 Prompt: Machine parameter
      mask DialogControl Container8 Prompt: Rotor
      mask DialogControl Container9 Prompt: Machine
      mask DialogControl Container10 Prompt: parameter
      mask DialogControl Container11 Prompt: inital value
      mask DialogControl Container12 Prompt: Rotor side control
      mask DialogControl Container13 Prompt: Control parameter
      mask DialogControl Container14 Prompt: Initial value
      mask DialogControl Container15 Prompt: reactive power
      mask DialogControl Container16 Prompt: Grid side control
      mask DialogControl Container17 Prompt: parameter
      mask DialogControl Container18 Prompt: reference
      mask DialogControl Container19 Prompt: inital value
      mask DialogControl Container20 Prompt: converter function
      mask DialogControl Container21 Prompt: inital value
      mask DialogControl Container22 Prompt: DC function
  Ixy : Outport
  wires:
  ES1/2(isxy) -> Mux4/1
  ES1/3(GBxy) -> Mux4/2
  Generator1/2(Igxy1) -> Mux6/1
  Generator1/3(GBxy) -> Mux6/2
  Mux4/1 -> Mux3/1
  Mux1/1 -> Mux3/2
  Mux2/1 -> Mux3/3
  Mux5/1 -> Mux3/4
  Mux6/1 -> Mux3/5
  Demux1/1 -> ES1/1(us_xy)
  Demux1/2 -> ES2/1(us_xy)
  Wind Generator - DFIG3/2(Igxy1) -> Mux7/1
  Wind Generator - DFIG3/3(GBxy) -> Mux7/2
  Wind Generator - DFIG4/2(Igxy1) -> Mux8/1
  Wind Generator - DFIG4/3(GBxy) -> Mux8/2
  Generator3/2(Igxy1) -> Mux11/1
  Generator3/3(GBxy) -> Mux11/2
  ES3/2(isxy) -> Mux12/1
  ES3/3(GBxy) -> Mux12/2
  Mux10/1 -> Mux9/1
  Mux7/1 -> Mux9/2
  Mux8/1 -> Mux9/3
  Mux11/1 -> Mux9/4
  Mux12/1 -> Mux9/5
  Mux13/1 -> Ixy/1
  Mux9/1 -> Mux13/2
  Mux3/1 -> Mux13/1
  Vxy/1 -> Demux/1
  Demux/1 -> Demux1/1
  Demux/2 -> Demux2/1
  Demux/3 -> [Vn], Scope10/1
  ES2/2(isxy) -> Mux1/1
  ES2/3(GBxy) -> Mux1/2
  ES1/1(m) -> [G1]
  ES2/1(m) -> [G2]
  Generator1/1(m) -> [G5]
  Wind Generator - DFIG3/1(m) -> [G7]
  Wind Generator - DFIG4/1(m) -> [G8]
  Generator3/1(m) -> [G9]
  ES3/1(m) -> [G10]
  [G1] -> Bus Selector/1
  Bus Selector/1 -> Scope/1  "<w>"
  [G8] -> Bus Selector27/1
  [G1] -> Bus Selector20/1
  [G2] -> Bus Selector21/1
  [G7] -> Bus Selector26/1
  [G10] -> Bus Selector29/1
  [G9] -> Bus Selector28/1
  [G4] -> Bus Selector23/1
  [G3] -> Bus Selector22/1
  [G6] -> Bus Selector25/1
  [G5] -> Bus Selector24/1
  Bus Selector20/1 -> Scope2/1  "<Pe>"
  Bus Selector21/1 -> Scope2/2  "<Pe>"
  Bus Selector22/1 -> Scope2/3  "<Pwind>"
  Bus Selector23/1 -> Scope2/4  "<Pwind>"
  Bus Selector24/1 -> Scope2/5  "<Pe>"
  Bus Selector25/1 -> Scope2/6  "<Pe>"
  Bus Selector28/1 -> Scope3/1  "<Pe>"
  Bus Selector29/1 -> Scope3/2  "<Pe>"
  [G2] -> Bus Selector1/1
  Bus Selector1/1 -> Scope/2  "<w>"
  [G3] -> Bus Selector2/1
  Bus Selector2/1 -> Scope/3  "<fw>"
  [G4] -> Bus Selector3/1
  Bus Selector3/1 -> Scope/4  "<fw>"
  [G5] -> Bus Selector4/1
  Bus Selector4/1 -> Scope/5  "<f>"
  [G6] -> Bus Selector5/1
  Bus Selector5/1 -> Scope/6  "<f>"
  [G10] -> Bus Selector9/1
  Bus Selector9/1 -> Scope1/2  "<w>"
  [G9] -> Bus Selector6/1
  Bus Selector6/1 -> Scope1/1  "<f>"
  [ROCOF_ES] -> Gain17/1
  Mux24/1 -> Scope16/1  "Sim2Python"
  Gain17/1 -> Scope5/1, Mux24/3
  Mux14/1 -> Mux24/1
  Gain/1 -> Mux24/2, Scope4/1
  Bus Selector19/1 -> Mux14/6  "<Pe>"
  [G6] -> Bus Selector19/1
  Bus Selector17/1 -> Mux14/4  "<fw>"
  Bus Selector18/1 -> Mux14/5  "<Pe>"
  [G2] -> Bus Selector15/1
  Bus Selector15/1 -> Mux14/2  "<Pe>"
  Bus Selector14/1 -> Mux14/1  "<Pe>"
  [G4] -> Bus Selector17/1
  [G5] -> Bus Selector18/1
  Bus Selector16/1 -> Mux14/3  "<fw>"
  [G1] -> Bus Selector14/1
  [G3] -> Bus Selector16/1
  [G7] -> Bus Selector10/1
  [G8] -> Bus Selector11/1
  Bus Selector10/1 -> Mux14/7  "<fw>"
  Bus Selector11/1 -> Mux14/8  "<fw>"
  W_ES/1(W_ES) -> Goto11/1
  [W_ES] -> Gain/1
  ROCOF_ES/1(ROCOF_ES) -> Goto12/1
  [deltaHess1] -> Sum/1
  Sum3/1 -> Sum4/1
  [deltaHess4] -> Sum1/2
  Sum/1 -> Sum3/1
  [deltaHess6] -> Sum2/2
  [deltaDess1] -> Sum5/1
  [deltaDess5] -> Sum7/1
  Sum1/1 -> Sum3/2
  Sum7/1 -> Sum9/2
  [deltaDess4] -> Sum6/2
  [deltaDess3] -> Sum6/1
  Sum8/1 -> Sum9/1
  Sum2/1 -> Sum4/2
  Sum5/1 -> Sum8/1
  [deltaHess2] -> Sum/2
  [deltaDess2] -> Sum5/2
  [deltaHess3] -> Sum1/1
  [deltaHess5] -> Sum2/1
  [deltaDess6] -> Sum7/2
  Sum6/1 -> Sum8/2
  [deltaHess7] -> Sum10/1
  Sum10/1 -> Sum11/2
  [deltaHess8] -> Sum10/2
  Sum11/1 -> Gain1/1
  Sum4/1 -> Sum11/1
  Gain1/1 -> Gain3/1
  Sum9/1 -> Sum12/1
  Sum12/1 -> Gain2/1
  [deltaDess8] -> Sum13/2
  [deltaDess7] -> Sum13/1
  Sum13/1 -> Sum12/2
  Gain2/1 -> Gain4/1
  Gain3/1 -> [Hess_avg]
  Gain4/1 -> [Dess_avg]
  [Hess_avg] -> Scope6/1, Mux24/4
  [Dess_avg] -> Scope7/1, Mux24/5
  [G7] -> Bus Selector7/1
  Bus Selector7/1 -> Scope/7  "<fw>"
  [G8] -> Bus Selector8/1
  Bus Selector8/1 -> Scope/8  "<fw>"
  Bus Selector26/1 -> Scope2/7  "<Pwind>"
  Bus Selector27/1 -> Scope2/8  "<Pwind>"
  Mux15/1 -> Gain19/1
  Add2/1 -> Gain18/1  "Pess1"
  [WreES1] -> Mux15/1  "W1"
  Integrator/1 -> Scope8/1  "L2norm"
  Gain18/1 -> Add/2
  Add/1 -> Product/2, Math Function/1
  Product/1 -> Integrator/1
  Gain19/1 -> Add/1, Add2/1
  Math Function/1 -> Product/1
  [WreES2] -> Mux15/2  "W2"
  [WreES4] -> Mux15/4  "W4"
  [WreES3] -> Mux15/3  "W3"
  [WreES5] -> Mux15/5  "W5"
  [WreES6] -> Mux15/6  "W6"
  [WreES7] -> Mux15/7  "W7"
  [WreES8] -> Mux15/8  "W8"
  Wind Generator - DFIG1/1(m) -> [G3]
  Wind Generator - DFIG1/2(Igxy1) -> Mux2/1
  Wind Generator - DFIG1/3(GBxy) -> Mux2/2
  Demux1/4 -> Wind Generator - DFIG2/2(Vsxy)
  Demux1/3 -> Wind Generator - DFIG1/2(Vsxy)
  Wind Generator - DFIG2/1(m) -> [G4]
  Wind Generator - DFIG2/2(Igxy1) -> Mux5/1
  Wind Generator - DFIG2/3(GBxy) -> Mux5/2
  Generator2/1(m) -> [G6]
  Generator2/2(Igxy1) -> Mux10/1
  Generator2/3(GBxy) -> Mux10/2
  Demux2/2 -> Wind Generator - DFIG3/2(Vsxy)
  Demux2/3 -> Wind Generator - DFIG4/2(Vsxy)
  Demux2/5 -> ES3/1(us_xy)
  Demux2/6 -> Generator4/1(Vgxy)
  Generator4/2(Igxy1) -> Mux16/1
  Generator4/3(GBxy) -> Mux16/2
  Mux16/1 -> Mux9/6
  Generator4/1(m) -> [G11]
  Generator5/3(GBxy) -> Mux17/2
  Generator5/2(Igxy1) -> Mux17/1
  Generator5/1(m) -> [G12]
  Mux17/1 -> Mux9/7
  Demux2/7 -> Generator5/1(Vgxy)
  Demux1/5 -> Generator1/1(Vgxy)
  Demux2/1 -> Generator2/1(Vgxy)
  Demux2/4 -> Generator3/1(Vgxy)
  Constant/1 -> Wind Generator - DFIG1/1(Wind speed)
  Constant1/1 -> Wind Generator - DFIG2/1(Wind speed)
  Constant2/1 -> Wind Generator - DFIG3/1(Wind speed)
  Constant3/1 -> Wind Generator - DFIG4/1(Wind speed)

== system M10B39_es_V1/Network1 ==
  Ixy : Inport
  Assertion : Assertion  AssertionFailFcn=set_param(bdroot, 'SimulationCommand', 'pause')  StopWhenAssertionFail=off
  Clock : Clock
  Clock1 : Clock
  Constant : Constant  Value=0.001
  Mux : Mux  Inputs=2
  Relational Operator : RelationalOperator  Operator=<=  OutDataTypeStr=boolean  RndMeth=Simplest  InputSameDT=off
  Relational Operator1 : RelationalOperator  Operator=<=  OutDataTypeStr=boolean  RndMeth=Simplest  InputSameDT=off
  S-Function : S-Function  FunctionName=TS_net_1_new  Parameters=YY_load,ng  SFunctionDeploymentMode=off  EnableBusSupport=off
  S-Function Examples : simulink/User-Defined Functions/S-Function Examples  Commented=on
  S-Function1 : S-Function  Commented=on  Parameters=YY_load,ng  SFunctionDeploymentMode=off  EnableBusSupport=off
  Scope : Scope
  Sum : Sum  Inputs=|++
  pause_time : Constant  Value=100
  Vxy : Outport
  wires:
  Ixy/1 -> Mux/2
  Mux/1 -> S-Function/1
  S-Function/1 -> Vxy/1
  Clock/1 -> Relational Operator/1, Mux/1
  Relational Operator/1 -> Assertion/1
  Clock1/1 -> Relational Operator1/1
  pause_time/1 -> Sum/1, Relational Operator/2
  Sum/1 -> Relational Operator1/2
  Relational Operator1/1 -> Scope/1
  Constant/1 -> Sum/2
